simulink model "bai3"  (R2017b)
settings: Solver=FixedStepAuto  StartTime=0.0  StopTime=10.0  FixedStep=0.1  RelTol=1e-3
libraries: simulink x1
settings Model: Creator=ADMIN  LastModifiedBy=ADMIN

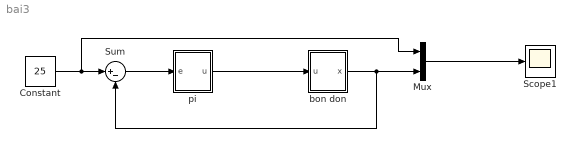
== system bai3 ==
  Constant : Constant  Value=25
  Mux : Mux  Inputs=2
  Scope1 : Scope
  Sum : Sum  Inputs=|+-
  bon don : Subsystem  mask{a=1, Cd=0.8, k=150, g=9.81, xdot=0, A_1=100}
      mask prompts: a "a="; Cd "Cd="; k "k="; g "g="; A_1 "A="
  "pi " : Subsystem  mask{kp=1, ki=0.0032, kd=0.01, T=0.1}
      mask prompts: kp "kp="; ki "ki="; kd "kd="; T "T="
  wires:
  Constant/1 -> Mux/1, Sum/1
  Sum/1 -> "pi "/1(e)
  bon don/1(x) -> Sum/2, Mux/2
  "pi "/1(u) -> bon don/1(u)
  Mux/1 -> Scope1/1

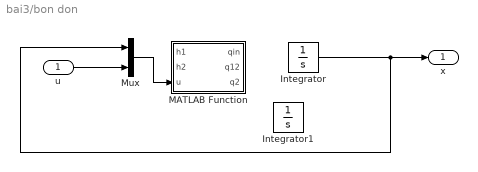
== system bai3/bon don ==
  u : Inport
  Integrator : Integrator  InitialCondition=xdot
  Integrator1 : Integrator  InitialCondition=xdot
  MATLAB Function : MATLAB Function  TreatAsAtomicUnit=on
  Mux : Mux  Inputs=2
  x : Outport
  wires:
  Integrator/1 -> Mux/1, x/1
  u/1 -> Mux/2
  Mux/1 -> MATLAB Function/3(u)

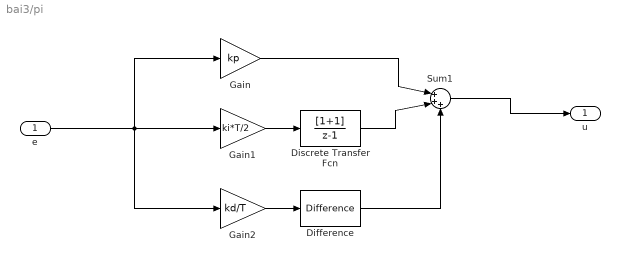
== system bai3/pi  ==
  e : Inport
  Difference : simulink/Discrete/Difference  ICPrevInput=0.0  OutMin=[]  OutMax=[]  OutDataType=fixdt(1, 16)  OutScaling=2^-10  DoSatur=off
  Discrete Transfer Fcn : DiscreteTransferFcn  Numerator=[1+1]  Denominator=[1 -1]
  Gain : Gain  Gain=kp
  Gain1 : Gain  Gain=ki*T/2
  Gain2 : Gain  Gain=kd/T
  Sum1 : Sum  Inputs=|+++
  u : Outport
  wires:
  e/1 -> Gain2/1, Gain1/1, Gain/1
  Sum1/1 -> u/1
  Gain1/1 -> Discrete Transfer Fcn/1
  Gain/1 -> Sum1/1
  Discrete Transfer Fcn/1 -> Sum1/2
  Difference/1 -> Sum1/3
  Gain2/1 -> Difference/1

== matlab function bai3/bon don/MATLAB Function ==
  data: h1 input; h2 input; u input; qin output; q12 output; q2 output
function [qin,q12,q2]=Flows(h1,h2,u)
%#codegen
C  = 0.6;  g  = 981;
b1 = 1.1;  b2 = 1.0;  K = 41;
qin  = K*u;
q12  = C*b1*sign(h1-h2)*sqrt(2*g*abs(h1-h2));
q2   = C*b2*sqrt(2*g*h2);
end
